simulink model "Dianlan_short"  (R2021a)
settings: Solver=VariableStepAuto  StartTime=0.0  StopTime=20e-6  RelTol=1e-3
libraries: spsGroundLib x4, spsVoltageMeasurementLib x3, spsDistributedParametersLineLib x2, spsSeriesRLCBranchLib x2, spsControlledVoltageSourceLib x1, spspowerguiLib x1
settings Model: Creator=张瑞  LastModifiedBy=张瑞

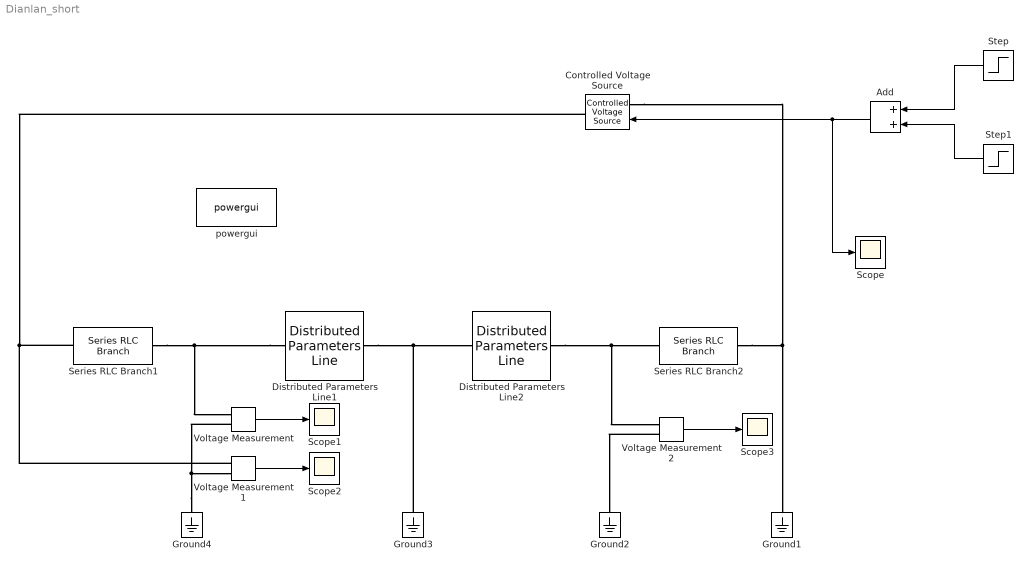
== system Dianlan_short ==
  Add : Sum
  Controlled Voltage Source : spsControlledVoltageSourceLib/Controlled Voltage Source  Initialize=off  Source_Type=AC  Amplitude=0  Phase=0  Frequency=0  Measurements=Voltage
  Distributed Parameters Line1 : spsDistributedParametersLineLib/Distributed Parameters Line  Phases=1  Length=1  Frequency=1000  Resistance=1.8E-1  Inductance=2.75E-4  Capacitance=5.57E-7  x1=[-1.238e-05 0;-1.237e-05 0;-1.236e-05 0;-1.235e-05 0;-1.234e-05 0;-1.233e-05 0;-1.232e-05 0;-1.231e-05 0;-1.23e-05 0;-1.229e-05 0;-1.228e-05 0;-1.227e-05 0;-1.226e-05 0;-1.225e-05 0;-1.224e-05 0;-1.223e-05 0;-1.222e-05 0;-1.221e-05 0;-1.22e-05 0;-1.219e-05 0;-1.218e-05 0;-1.217e-05 0;-1.216e-05 0;-1.215e-05 0;-1.214e-05 0;-1.213e-05 0;-1.212e-05 0;-1.211e-05 0;-1.21e-05 0;-1.209e-05 0;-1.208e-05 0;-1.207e-05 0;-1.206e-05 0;-1.205e-05 0;-1.204e-05 0;-1.203e-05 0;-1.202e-05 0;-1.201e-05 0;-1.2e-05 0;-1.199e-05 0;-1.198e-05 0;-1.197e-05 0;-1.196e-05 0;-1.195e-05 0;-1.194e-05 0;-1.193e-05 0;-1.192e-05 0;-1.191e-05 0;-1.19e-05 0;-1.189e-05 0;-1.188e-05 0;-1.187e-05 0;-1.186e-05 0;-1.185e-05 0;-1.184e-05 0;-1.183e-05 0;-1.182e-05 0;-1.181e-05 0;-1.18e-05 0;-1.179e-05 0;-1.178e-05 0;-1.177e-05 0;-1.176e-05 0;-1.175e-05 0;-1.174e-05 0;-1.173e-05 0;-1.172e-05 0;-1.171e-05 0;-1.17e-05 0;-1.169e-05 0;-1.168e-05 0;-1.167e-05 0;-1.166e-05 0;-1.165e-05 0;-1.164e-05 0;-1.163e-05 0;-1.162e-05 0;-1.161e-05 0;-1.16e-05 0;-1.159e-05 0;-1.158e-05 0;-1.157e-05 0;-1.156e-05 0;-1.155e-05 0;-1.154e-05 0;-1.153e-05 0;-1.152e-05 0;-1.151e-05 0;-1.15e-05 0;-1.149e-05 0;-1.148e-05 0;-1.147e-05 0;-1.146e-05 0;-1.145e-05 0;-1.144e-05 0;-1.143e-05 0;-1.142e-05 0;-1.141e-05 0;-1.14e-05 0;-1.139e-05 0;-1.138e-05 0;-1.137e-05 0;-1.136e-05 0;-1.135e-05 0;-1.134e-05 0;-1.133e-05 0;-1.132e-05 0;-1.131e-05 0;-1.13e-05 0;-1.129e-05 0;-1.128e-05 0;-1.127e-05 0;-1.126e-05 0;-1.125e-05 0;-1.124e-05 0;-1.123e-05 0;-1.122e-05 0;-1.121e-05 0;-1.12e-05 0;-1.119e-05 0;-1.118e-05 0;-1.117e-05 0;-1.116e-05 0;-1.115e-05 0;-1.114e-05 0;-1.113e-05 0;-1.112e-05 0;-1.111e-05 0;-1.11e-05 0;-1.109e-05 0;-1.108e-05 0;-1.107e-05 0;-1.106e-05 0;-1.105e-05 0;-1.104e-05 0;-1.103e-05 0;-1.102e-05 0;-1.101e-05 0;-1.1e-05 0;-1.099e-05 0;-1.098e-05 0;-1.097e-05 0;-1.096e-05 0;-1.095e-05 0;-1.094e-05 0;-1.093e-05 0;-1.092e-05 0;-1.091e-05 0;-1.09e-05 0;-1.089e-05 0;-1.088e-05 0;-1.087e-05 0;-1.086e-05 0;-1.085e-05 0;-1.084e-05 0;-1.083e-05 0;-1.082e-05 0;-1.081e-05 0;-1.08e-05 0;-1.079e-05 0;-1.078e-05 0;-1.077e-05 0;-1.076e-05 0;-1.075e-05 0;-1.074e-05 0;-1.073e-05 0;-1.072e-05 0;-1.071e-05 0;-1.07e-05 0;-1.069e-05 0;-1.068e-05 0;-1.067e-05 0;-1.066e-05 0;-1.065e-05 0;-1.064e-05 0;-1.063e-05 0;-1.062e-05 0;-1.061e-05 0;-1.06e-05 0;-1.059e-05 0;-1.058e-05 0;-1.057e-05 0;-1.056e-05 0;-1.055e-05 0;-1.054e-05 0;-1.053e-05 0;-1.052e-05 0;-1.051e-05 0;-1.05e-05 0;-1.049e-05 0;-1.048e-05 0;-1.047e-05 0;-1.046e-05 0;-1.045e-05 0;-1.044e-05 0;-1.043e-05 0;-1.042e-05 0;-1.041e-05 0;-1.04e-05 0;-1.039e-05 0;-1.038e-05 0;-1.037e-05 0;-1.036e-05 0;-1.035e-05 0;-1.034e-05 0;-1.033e-05 0;-1.032e-05 0;-1.031e-05 0;-1.03e-05 0;-1.029e-05 0;-1.028e-05 0;-1.027e-05 0;-1.026e-05 0;-1.025e-05 0;-1.024e-05 0;-1.023e-05 0;-1.022e-05 0;-1.021e-05 0;-1.02e-05 0;-1.019e-05 0;-1.018e-05 0;-1.017e-05 0;-1.016e-05 0;-1.015e-05 0;-1.014e-05 0;-1.013e-05 0;-1.012e-05 0;-1.011e-05 0;-1.01e-05 0;-1.009e-05 0;-1.008e-05 0;-1.007e-05 0;-1.006e-05 0;-1.005e-05 0;-1.004e-05 0;-1.003e-05 0;-1.002e-05 0;-1.001e-05 0;-1e-05 0;-9.99e-06 0;-9.98e-06 0;-9.97e-06 0;-9.96e-06 0;-9.95e-06 0;-9.94e-06 0;-9.93e-06 0;-9.92e-06 0;-9.91e-06 0;-9.9e-06 0;-9.89e-06 0;-9.88e-06 0;-9.87e-06 0;-9.86e-06 0;-9.85e-06 0;-9.84e-06 0;-9.83e-06 0;-9.82e-06 0;-9.81e-06 0;-9.8e-06 0;-9.79e-06 0;-9.78e-06 0;-9.77e-06 0;-9.76e-06 0;-9.75e-06 0;-9.74e-06 0;-9.73e-06 0;-9.72e-06 0;-9.71e-06 0;-9.7e-06 0;-9.69e-06 0;-9.68e-06 0;-9.67e-06 0;-9.66e-06 0;-9.65e-06 0;-9.64e-06 0;-9.63e-06 0;-9.62e-06 0;-9.61e-06 0;-9.6e-06 0;-9.59e-06 0;-9.58e-06 0;-9.57e-06 0;-9.56e-06 0;-9.55e-06 0;-9.54e-06 0;-9.53e-06 0;-9.52e-06 0;-9.51e-06 0;-9.5e-06 0;-9.49e-06 0;-9.48e-06 0;-9.47e-06 0;-9.46e-06 0;-9.45e-06 0;-9.44e-06 0;-9.43e-06 0;-9.42e-06 0;-9.41e-06 0;-9.4e-06 0;-9.39e-06 0;-9.38e-06 0;-9.37e-06 0;-9.36e-06 0;-9.35e-06 0;-9.34e-06 0;-9.33e-06 0;-9.32e-06 0;-9.31e-06 0;-9.3e-06 0;-9.29e-06 0;-9.28e-06 0;-9.27e-06 0;-9.26e-06 0;-9.25e-06 0;-9.24e-06 0;-9.23e-06 0 ...(+10828 chars)]  x2=[-1.238e-05 0;-1.237e-05 0;-1.236e-05 0;-1.235e-05 0;-1.234e-05 0;-1.233e-05 0;-1.232e-05 0;-1.231e-05 0;-1.23e-05 0;-1.229e-05 0;-1.228e-05 0;-1.227e-05 0;-1.226e-05 0;-1.225e-05 0;-1.224e-05 0;-1.223e-05 0;-1.222e-05 0;-1.221e-05 0;-1.22e-05 0;-1.219e-05 0;-1.218e-05 0;-1.217e-05 0;-1.216e-05 0;-1.215e-05 0;-1.214e-05 0;-1.213e-05 0;-1.212e-05 0;-1.211e-05 0;-1.21e-05 0;-1.209e-05 0;-1.208e-05 0;-1.207e-05 0;-1.206e-05 0;-1.205e-05 0;-1.204e-05 0;-1.203e-05 0;-1.202e-05 0;-1.201e-05 0;-1.2e-05 0;-1.199e-05 0;-1.198e-05 0;-1.197e-05 0;-1.196e-05 0;-1.195e-05 0;-1.194e-05 0;-1.193e-05 0;-1.192e-05 0;-1.191e-05 0;-1.19e-05 0;-1.189e-05 0;-1.188e-05 0;-1.187e-05 0;-1.186e-05 0;-1.185e-05 0;-1.184e-05 0;-1.183e-05 0;-1.182e-05 0;-1.181e-05 0;-1.18e-05 0;-1.179e-05 0;-1.178e-05 0;-1.177e-05 0;-1.176e-05 0;-1.175e-05 0;-1.174e-05 0;-1.173e-05 0;-1.172e-05 0;-1.171e-05 0;-1.17e-05 0;-1.169e-05 0;-1.168e-05 0;-1.167e-05 0;-1.166e-05 0;-1.165e-05 0;-1.164e-05 0;-1.163e-05 0;-1.162e-05 0;-1.161e-05 0;-1.16e-05 0;-1.159e-05 0;-1.158e-05 0;-1.157e-05 0;-1.156e-05 0;-1.155e-05 0;-1.154e-05 0;-1.153e-05 0;-1.152e-05 0;-1.151e-05 0;-1.15e-05 0;-1.149e-05 0;-1.148e-05 0;-1.147e-05 0;-1.146e-05 0;-1.145e-05 0;-1.144e-05 0;-1.143e-05 0;-1.142e-05 0;-1.141e-05 0;-1.14e-05 0;-1.139e-05 0;-1.138e-05 0;-1.137e-05 0;-1.136e-05 0;-1.135e-05 0;-1.134e-05 0;-1.133e-05 0;-1.132e-05 0;-1.131e-05 0;-1.13e-05 0;-1.129e-05 0;-1.128e-05 0;-1.127e-05 0;-1.126e-05 0;-1.125e-05 0;-1.124e-05 0;-1.123e-05 0;-1.122e-05 0;-1.121e-05 0;-1.12e-05 0;-1.119e-05 0;-1.118e-05 0;-1.117e-05 0;-1.116e-05 0;-1.115e-05 0;-1.114e-05 0;-1.113e-05 0;-1.112e-05 0;-1.111e-05 0;-1.11e-05 0;-1.109e-05 0;-1.108e-05 0;-1.107e-05 0;-1.106e-05 0;-1.105e-05 0;-1.104e-05 0;-1.103e-05 0;-1.102e-05 0;-1.101e-05 0;-1.1e-05 0;-1.099e-05 0;-1.098e-05 0;-1.097e-05 0;-1.096e-05 0;-1.095e-05 0;-1.094e-05 0;-1.093e-05 0;-1.092e-05 0;-1.091e-05 0;-1.09e-05 0;-1.089e-05 0;-1.088e-05 0;-1.087e-05 0;-1.086e-05 0;-1.085e-05 0;-1.084e-05 0;-1.083e-05 0;-1.082e-05 0;-1.081e-05 0;-1.08e-05 0;-1.079e-05 0;-1.078e-05 0;-1.077e-05 0;-1.076e-05 0;-1.075e-05 0;-1.074e-05 0;-1.073e-05 0;-1.072e-05 0;-1.071e-05 0;-1.07e-05 0;-1.069e-05 0;-1.068e-05 0;-1.067e-05 0;-1.066e-05 0;-1.065e-05 0;-1.064e-05 0;-1.063e-05 0;-1.062e-05 0;-1.061e-05 0;-1.06e-05 0;-1.059e-05 0;-1.058e-05 0;-1.057e-05 0;-1.056e-05 0;-1.055e-05 0;-1.054e-05 0;-1.053e-05 0;-1.052e-05 0;-1.051e-05 0;-1.05e-05 0;-1.049e-05 0;-1.048e-05 0;-1.047e-05 0;-1.046e-05 0;-1.045e-05 0;-1.044e-05 0;-1.043e-05 0;-1.042e-05 0;-1.041e-05 0;-1.04e-05 0;-1.039e-05 0;-1.038e-05 0;-1.037e-05 0;-1.036e-05 0;-1.035e-05 0;-1.034e-05 0;-1.033e-05 0;-1.032e-05 0;-1.031e-05 0;-1.03e-05 0;-1.029e-05 0;-1.028e-05 0;-1.027e-05 0;-1.026e-05 0;-1.025e-05 0;-1.024e-05 0;-1.023e-05 0;-1.022e-05 0;-1.021e-05 0;-1.02e-05 0;-1.019e-05 0;-1.018e-05 0;-1.017e-05 0;-1.016e-05 0;-1.015e-05 0;-1.014e-05 0;-1.013e-05 0;-1.012e-05 0;-1.011e-05 0;-1.01e-05 0;-1.009e-05 0;-1.008e-05 0;-1.007e-05 0;-1.006e-05 0;-1.005e-05 0;-1.004e-05 0;-1.003e-05 0;-1.002e-05 0;-1.001e-05 0;-1e-05 0;-9.99e-06 0;-9.98e-06 0;-9.97e-06 0;-9.96e-06 0;-9.95e-06 0;-9.94e-06 0;-9.93e-06 0;-9.92e-06 0;-9.91e-06 0;-9.9e-06 0;-9.89e-06 0;-9.88e-06 0;-9.87e-06 0;-9.86e-06 0;-9.85e-06 0;-9.84e-06 0;-9.83e-06 0;-9.82e-06 0;-9.81e-06 0;-9.8e-06 0;-9.79e-06 0;-9.78e-06 0;-9.77e-06 0;-9.76e-06 0;-9.75e-06 0;-9.74e-06 0;-9.73e-06 0;-9.72e-06 0;-9.71e-06 0;-9.7e-06 0;-9.69e-06 0;-9.68e-06 0;-9.67e-06 0;-9.66e-06 0;-9.65e-06 0;-9.64e-06 0;-9.63e-06 0;-9.62e-06 0;-9.61e-06 0;-9.6e-06 0;-9.59e-06 0;-9.58e-06 0;-9.57e-06 0;-9.56e-06 0;-9.55e-06 0;-9.54e-06 0;-9.53e-06 0;-9.52e-06 0;-9.51e-06 0;-9.5e-06 0;-9.49e-06 0;-9.48e-06 0;-9.47e-06 0;-9.46e-06 0;-9.45e-06 0;-9.44e-06 0;-9.43e-06 0;-9.42e-06 0;-9.41e-06 0;-9.4e-06 0;-9.39e-06 0;-9.38e-06 0;-9.37e-06 0;-9.36e-06 0;-9.35e-06 0;-9.34e-06 0;-9.33e-06 0;-9.32e-06 0;-9.31e-06 0;-9.3e-06 0;-9.29e-06 0;-9.28e-06 0;-9.27e-06 0;-9.26e-06 0;-9.25e-06 0;-9.24e-06 0;-9.23e-06 0 ...(+10828 chars)]  x3=[-1.238e-05 0;-1.237e-05 0;-1.236e-05 0;-1.235e-05 0;-1.234e-05 0;-1.233e-05 0;-1.232e-05 0;-1.231e-05 0;-1.23e-05 0;-1.229e-05 0;-1.228e-05 0;-1.227e-05 0;-1.226e-05 0;-1.225e-05 0;-1.224e-05 0;-1.223e-05 0;-1.222e-05 0;-1.221e-05 0;-1.22e-05 0;-1.219e-05 0;-1.218e-05 0;-1.217e-05 0;-1.216e-05 0;-1.215e-05 0;-1.214e-05 0;-1.213e-05 0;-1.212e-05 0;-1.211e-05 0;-1.21e-05 0;-1.209e-05 0;-1.208e-05 0;-1.207e-05 0;-1.206e-05 0;-1.205e-05 0;-1.204e-05 0;-1.203e-05 0;-1.202e-05 0;-1.201e-05 0;-1.2e-05 0;-1.199e-05 0;-1.198e-05 0;-1.197e-05 0;-1.196e-05 0;-1.195e-05 0;-1.194e-05 0;-1.193e-05 0;-1.192e-05 0;-1.191e-05 0;-1.19e-05 0;-1.189e-05 0;-1.188e-05 0;-1.187e-05 0;-1.186e-05 0;-1.185e-05 0;-1.184e-05 0;-1.183e-05 0;-1.182e-05 0;-1.181e-05 0;-1.18e-05 0;-1.179e-05 0;-1.178e-05 0;-1.177e-05 0;-1.176e-05 0;-1.175e-05 0;-1.174e-05 0;-1.173e-05 0;-1.172e-05 0;-1.171e-05 0;-1.17e-05 0;-1.169e-05 0;-1.168e-05 0;-1.167e-05 0;-1.166e-05 0;-1.165e-05 0;-1.164e-05 0;-1.163e-05 0;-1.162e-05 0;-1.161e-05 0;-1.16e-05 0;-1.159e-05 0;-1.158e-05 0;-1.157e-05 0;-1.156e-05 0;-1.155e-05 0;-1.154e-05 0;-1.153e-05 0;-1.152e-05 0;-1.151e-05 0;-1.15e-05 0;-1.149e-05 0;-1.148e-05 0;-1.147e-05 0;-1.146e-05 0;-1.145e-05 0;-1.144e-05 0;-1.143e-05 0;-1.142e-05 0;-1.141e-05 0;-1.14e-05 0;-1.139e-05 0;-1.138e-05 0;-1.137e-05 0;-1.136e-05 0;-1.135e-05 0;-1.134e-05 0;-1.133e-05 0;-1.132e-05 0;-1.131e-05 0;-1.13e-05 0;-1.129e-05 0;-1.128e-05 0;-1.127e-05 0;-1.126e-05 0;-1.125e-05 0;-1.124e-05 0;-1.123e-05 0;-1.122e-05 0;-1.121e-05 0;-1.12e-05 0;-1.119e-05 0;-1.118e-05 0;-1.117e-05 0;-1.116e-05 0;-1.115e-05 0;-1.114e-05 0;-1.113e-05 0;-1.112e-05 0;-1.111e-05 0;-1.11e-05 0;-1.109e-05 0;-1.108e-05 0;-1.107e-05 0;-1.106e-05 0;-1.105e-05 0;-1.104e-05 0;-1.103e-05 0;-1.102e-05 0;-1.101e-05 0;-1.1e-05 0;-1.099e-05 0;-1.098e-05 0;-1.097e-05 0;-1.096e-05 0;-1.095e-05 0;-1.094e-05 0;-1.093e-05 0;-1.092e-05 0;-1.091e-05 0;-1.09e-05 0;-1.089e-05 0;-1.088e-05 0;-1.087e-05 0;-1.086e-05 0;-1.085e-05 0;-1.084e-05 0;-1.083e-05 0;-1.082e-05 0;-1.081e-05 0;-1.08e-05 0;-1.079e-05 0;-1.078e-05 0;-1.077e-05 0;-1.076e-05 0;-1.075e-05 0;-1.074e-05 0;-1.073e-05 0;-1.072e-05 0;-1.071e-05 0;-1.07e-05 0;-1.069e-05 0;-1.068e-05 0;-1.067e-05 0;-1.066e-05 0;-1.065e-05 0;-1.064e-05 0;-1.063e-05 0;-1.062e-05 0;-1.061e-05 0;-1.06e-05 0;-1.059e-05 0;-1.058e-05 0;-1.057e-05 0;-1.056e-05 0;-1.055e-05 0;-1.054e-05 0;-1.053e-05 0;-1.052e-05 0;-1.051e-05 0;-1.05e-05 0;-1.049e-05 0;-1.048e-05 0;-1.047e-05 0;-1.046e-05 0;-1.045e-05 0;-1.044e-05 0;-1.043e-05 0;-1.042e-05 0;-1.041e-05 0;-1.04e-05 0;-1.039e-05 0;-1.038e-05 0;-1.037e-05 0;-1.036e-05 0;-1.035e-05 0;-1.034e-05 0;-1.033e-05 0;-1.032e-05 0;-1.031e-05 0;-1.03e-05 0;-1.029e-05 0;-1.028e-05 0;-1.027e-05 0;-1.026e-05 0;-1.025e-05 0;-1.024e-05 0;-1.023e-05 0;-1.022e-05 0;-1.021e-05 0;-1.02e-05 0;-1.019e-05 0;-1.018e-05 0;-1.017e-05 0;-1.016e-05 0;-1.015e-05 0;-1.014e-05 0;-1.013e-05 0;-1.012e-05 0;-1.011e-05 0;-1.01e-05 0;-1.009e-05 0;-1.008e-05 0;-1.007e-05 0;-1.006e-05 0;-1.005e-05 0;-1.004e-05 0;-1.003e-05 0;-1.002e-05 0;-1.001e-05 0;-1e-05 0;-9.99e-06 0;-9.98e-06 0;-9.97e-06 0;-9.96e-06 0;-9.95e-06 0;-9.94e-06 0;-9.93e-06 0;-9.92e-06 0;-9.91e-06 0;-9.9e-06 0;-9.89e-06 0;-9.88e-06 0;-9.87e-06 0;-9.86e-06 0;-9.85e-06 0;-9.84e-06 0;-9.83e-06 0;-9.82e-06 0;-9.81e-06 0;-9.8e-06 0;-9.79e-06 0;-9.78e-06 0;-9.77e-06 0;-9.76e-06 0;-9.75e-06 0;-9.74e-06 0;-9.73e-06 0;-9.72e-06 0;-9.71e-06 0;-9.7e-06 0;-9.69e-06 0;-9.68e-06 0;-9.67e-06 0;-9.66e-06 0;-9.65e-06 0;-9.64e-06 0;-9.63e-06 0;-9.62e-06 0;-9.61e-06 0;-9.6e-06 0;-9.59e-06 0;-9.58e-06 0;-9.57e-06 0;-9.56e-06 0;-9.55e-06 0;-9.54e-06 0;-9.53e-06 0;-9.52e-06 0;-9.51e-06 0;-9.5e-06 0;-9.49e-06 0;-9.48e-06 0;-9.47e-06 0;-9.46e-06 0;-9.45e-06 0;-9.44e-06 0;-9.43e-06 0;-9.42e-06 0;-9.41e-06 0;-9.4e-06 0;-9.39e-06 0;-9.38e-06 0;-9.37e-06 0;-9.36e-06 0;-9.35e-06 0;-9.34e-06 0;-9.33e-06 0;-9.32e-06 0;-9.31e-06 0;-9.3e-06 0;-9.29e-06 0;-9.28e-06 0;-9.27e-06 0;-9.26e-06 0;-9.25e-06 0;-9.24e-06 0;-9.23e-06 0 ...(+10828 chars)]  x4=[-1.238e-05 0;-1.237e-05 0;-1.236e-05 0;-1.235e-05 0;-1.234e-05 0;-1.233e-05 0;-1.232e-05 0;-1.231e-05 0;-1.23e-05 0;-1.229e-05 0;-1.228e-05 0;-1.227e-05 0;-1.226e-05 0;-1.225e-05 0;-1.224e-05 0;-1.223e-05 0;-1.222e-05 0;-1.221e-05 0;-1.22e-05 0;-1.219e-05 0;-1.218e-05 0;-1.217e-05 0;-1.216e-05 0;-1.215e-05 0;-1.214e-05 0;-1.213e-05 0;-1.212e-05 0;-1.211e-05 0;-1.21e-05 0;-1.209e-05 0;-1.208e-05 0;-1.207e-05 0;-1.206e-05 0;-1.205e-05 0;-1.204e-05 0;-1.203e-05 0;-1.202e-05 0;-1.201e-05 0;-1.2e-05 0;-1.199e-05 0;-1.198e-05 0;-1.197e-05 0;-1.196e-05 0;-1.195e-05 0;-1.194e-05 0;-1.193e-05 0;-1.192e-05 0;-1.191e-05 0;-1.19e-05 0;-1.189e-05 0;-1.188e-05 0;-1.187e-05 0;-1.186e-05 0;-1.185e-05 0;-1.184e-05 0;-1.183e-05 0;-1.182e-05 0;-1.181e-05 0;-1.18e-05 0;-1.179e-05 0;-1.178e-05 0;-1.177e-05 0;-1.176e-05 0;-1.175e-05 0;-1.174e-05 0;-1.173e-05 0;-1.172e-05 0;-1.171e-05 0;-1.17e-05 0;-1.169e-05 0;-1.168e-05 0;-1.167e-05 0;-1.166e-05 0;-1.165e-05 0;-1.164e-05 0;-1.163e-05 0;-1.162e-05 0;-1.161e-05 0;-1.16e-05 0;-1.159e-05 0;-1.158e-05 0;-1.157e-05 0;-1.156e-05 0;-1.155e-05 0;-1.154e-05 0;-1.153e-05 0;-1.152e-05 0;-1.151e-05 0;-1.15e-05 0;-1.149e-05 0;-1.148e-05 0;-1.147e-05 0;-1.146e-05 0;-1.145e-05 0;-1.144e-05 0;-1.143e-05 0;-1.142e-05 0;-1.141e-05 0;-1.14e-05 0;-1.139e-05 0;-1.138e-05 0;-1.137e-05 0;-1.136e-05 0;-1.135e-05 0;-1.134e-05 0;-1.133e-05 0;-1.132e-05 0;-1.131e-05 0;-1.13e-05 0;-1.129e-05 0;-1.128e-05 0;-1.127e-05 0;-1.126e-05 0;-1.125e-05 0;-1.124e-05 0;-1.123e-05 0;-1.122e-05 0;-1.121e-05 0;-1.12e-05 0;-1.119e-05 0;-1.118e-05 0;-1.117e-05 0;-1.116e-05 0;-1.115e-05 0;-1.114e-05 0;-1.113e-05 0;-1.112e-05 0;-1.111e-05 0;-1.11e-05 0;-1.109e-05 0;-1.108e-05 0;-1.107e-05 0;-1.106e-05 0;-1.105e-05 0;-1.104e-05 0;-1.103e-05 0;-1.102e-05 0;-1.101e-05 0;-1.1e-05 0;-1.099e-05 0;-1.098e-05 0;-1.097e-05 0;-1.096e-05 0;-1.095e-05 0;-1.094e-05 0;-1.093e-05 0;-1.092e-05 0;-1.091e-05 0;-1.09e-05 0;-1.089e-05 0;-1.088e-05 0;-1.087e-05 0;-1.086e-05 0;-1.085e-05 0;-1.084e-05 0;-1.083e-05 0;-1.082e-05 0;-1.081e-05 0;-1.08e-05 0;-1.079e-05 0;-1.078e-05 0;-1.077e-05 0;-1.076e-05 0;-1.075e-05 0;-1.074e-05 0;-1.073e-05 0;-1.072e-05 0;-1.071e-05 0;-1.07e-05 0;-1.069e-05 0;-1.068e-05 0;-1.067e-05 0;-1.066e-05 0;-1.065e-05 0;-1.064e-05 0;-1.063e-05 0;-1.062e-05 0;-1.061e-05 0;-1.06e-05 0;-1.059e-05 0;-1.058e-05 0;-1.057e-05 0;-1.056e-05 0;-1.055e-05 0;-1.054e-05 0;-1.053e-05 0;-1.052e-05 0;-1.051e-05 0;-1.05e-05 0;-1.049e-05 0;-1.048e-05 0;-1.047e-05 0;-1.046e-05 0;-1.045e-05 0;-1.044e-05 0;-1.043e-05 0;-1.042e-05 0;-1.041e-05 0;-1.04e-05 0;-1.039e-05 0;-1.038e-05 0;-1.037e-05 0;-1.036e-05 0;-1.035e-05 0;-1.034e-05 0;-1.033e-05 0;-1.032e-05 0;-1.031e-05 0;-1.03e-05 0;-1.029e-05 0;-1.028e-05 0;-1.027e-05 0;-1.026e-05 0;-1.025e-05 0;-1.024e-05 0;-1.023e-05 0;-1.022e-05 0;-1.021e-05 0;-1.02e-05 0;-1.019e-05 0;-1.018e-05 0;-1.017e-05 0;-1.016e-05 0;-1.015e-05 0;-1.014e-05 0;-1.013e-05 0;-1.012e-05 0;-1.011e-05 0;-1.01e-05 0;-1.009e-05 0;-1.008e-05 0;-1.007e-05 0;-1.006e-05 0;-1.005e-05 0;-1.004e-05 0;-1.003e-05 0;-1.002e-05 0;-1.001e-05 0;-1e-05 0;-9.99e-06 0;-9.98e-06 0;-9.97e-06 0;-9.96e-06 0;-9.95e-06 0;-9.94e-06 0;-9.93e-06 0;-9.92e-06 0;-9.91e-06 0;-9.9e-06 0;-9.89e-06 0;-9.88e-06 0;-9.87e-06 0;-9.86e-06 0;-9.85e-06 0;-9.84e-06 0;-9.83e-06 0;-9.82e-06 0;-9.81e-06 0;-9.8e-06 0;-9.79e-06 0;-9.78e-06 0;-9.77e-06 0;-9.76e-06 0;-9.75e-06 0;-9.74e-06 0;-9.73e-06 0;-9.72e-06 0;-9.71e-06 0;-9.7e-06 0;-9.69e-06 0;-9.68e-06 0;-9.67e-06 0;-9.66e-06 0;-9.65e-06 0;-9.64e-06 0;-9.63e-06 0;-9.62e-06 0;-9.61e-06 0;-9.6e-06 0;-9.59e-06 0;-9.58e-06 0;-9.57e-06 0;-9.56e-06 0;-9.55e-06 0;-9.54e-06 0;-9.53e-06 0;-9.52e-06 0;-9.51e-06 0;-9.5e-06 0;-9.49e-06 0;-9.48e-06 0;-9.47e-06 0;-9.46e-06 0;-9.45e-06 0;-9.44e-06 0;-9.43e-06 0;-9.42e-06 0;-9.41e-06 0;-9.4e-06 0;-9.39e-06 0;-9.38e-06 0;-9.37e-06 0;-9.36e-06 0;-9.35e-06 0;-9.34e-06 0;-9.33e-06 0;-9.32e-06 0;-9.31e-06 0;-9.3e-06 0;-9.29e-06 0;-9.28e-06 0;-9.27e-06 0;-9.26e-06 0;-9.25e-06 0;-9.24e-06 0;-9.23e-06 0 ...(+10828 chars)]  x5=1.23763888109577e-05  V1=ones(3,3)  V2=ones(3,3)  I1=ones(3,3)  I2=ones(3,3)  nHarmo=1  Measurements=Phase-to-ground voltages  Decoupling=off  VsMag0=0  VrMag0=0  VsAngle0=0  VrAngle0=0  IsMag0=0  IrMag0=0  IsAngle0=0  IrAngle0=0
      settings: SourceProductBaseCode=PS
  Distributed Parameters Line2 : spsDistributedParametersLineLib/Distributed Parameters Line  Phases=1  Length=0.2  Frequency=1000  Resistance=1.8E-1  Inductance=2.75E-4  Capacitance=5.57E-7  x1=[-2.48e-06 0;-2.47e-06 0;-2.46e-06 0;-2.45e-06 0;-2.44e-06 0;-2.43e-06 0;-2.42e-06 0;-2.41e-06 0;-2.4e-06 0;-2.39e-06 0;-2.38e-06 0;-2.37e-06 0;-2.36e-06 0;-2.35e-06 0;-2.34e-06 0;-2.33e-06 0;-2.32e-06 0;-2.31e-06 0;-2.3e-06 0;-2.29e-06 0;-2.28e-06 0;-2.27e-06 0;-2.26e-06 0;-2.25e-06 0;-2.24e-06 0;-2.23e-06 0;-2.22e-06 0;-2.21e-06 0;-2.2e-06 0;-2.19e-06 0;-2.18e-06 0;-2.17e-06 0;-2.16e-06 0;-2.15e-06 0;-2.14e-06 0;-2.13e-06 0;-2.12e-06 0;-2.11e-06 0;-2.1e-06 0;-2.09e-06 0;-2.08e-06 0;-2.07e-06 0;-2.06e-06 0;-2.05e-06 0;-2.04e-06 0;-2.03e-06 0;-2.02e-06 0;-2.01e-06 0;-2e-06 0;-1.99e-06 0;-1.98e-06 0;-1.97e-06 0;-1.96e-06 0;-1.95e-06 0;-1.94e-06 0;-1.93e-06 0;-1.92e-06 0;-1.91e-06 0;-1.9e-06 0;-1.89e-06 0;-1.88e-06 0;-1.87e-06 0;-1.86e-06 0;-1.85e-06 0;-1.84e-06 0;-1.83e-06 0;-1.82e-06 0;-1.81e-06 0;-1.8e-06 0;-1.79e-06 0;-1.78e-06 0;-1.77e-06 0;-1.76e-06 0;-1.75e-06 0;-1.74e-06 0;-1.73e-06 0;-1.72e-06 0;-1.71e-06 0;-1.7e-06 0;-1.69e-06 0;-1.68e-06 0;-1.67e-06 0;-1.66e-06 0;-1.65e-06 0;-1.64e-06 0;-1.63e-06 0;-1.62e-06 0;-1.61e-06 0;-1.6e-06 0;-1.59e-06 0;-1.58e-06 0;-1.57e-06 0;-1.56e-06 0;-1.55e-06 0;-1.54e-06 0;-1.53e-06 0;-1.52e-06 0;-1.51e-06 0;-1.5e-06 0;-1.49e-06 0;-1.48e-06 0;-1.47e-06 0;-1.46e-06 0;-1.45e-06 0;-1.44e-06 0;-1.43e-06 0;-1.42e-06 0;-1.41e-06 0;-1.4e-06 0;-1.39e-06 0;-1.38e-06 0;-1.37e-06 0;-1.36e-06 0;-1.35e-06 0;-1.34e-06 0;-1.33e-06 0;-1.32e-06 0;-1.31e-06 0;-1.3e-06 0;-1.29e-06 0;-1.28e-06 0;-1.27e-06 0;-1.26e-06 0;-1.25e-06 0;-1.24e-06 0;-1.23e-06 0;-1.22e-06 0;-1.21e-06 0;-1.2e-06 0;-1.19e-06 0;-1.18e-06 0;-1.17e-06 0;-1.16e-06 0;-1.15e-06 0;-1.14e-06 0;-1.13e-06 0;-1.12e-06 0;-1.11e-06 0;-1.1e-06 0;-1.09e-06 0;-1.08e-06 0;-1.07e-06 0;-1.06e-06 0;-1.05e-06 0;-1.04e-06 0;-1.03e-06 0;-1.02e-06 0;-1.01e-06 0;-1e-06 0;-9.9e-07 0;-9.8e-07 0;-9.7e-07 0;-9.6e-07 0;-9.5e-07 0;-9.4e-07 0;-9.3e-07 0;-9.2e-07 0;-9.1e-07 0;-9e-07 0;-8.9e-07 0;-8.8e-07 0;-8.7e-07 0;-8.6e-07 0;-8.5e-07 0;-8.4e-07 0;-8.3e-07 0;-8.2e-07 0;-8.1e-07 0;-8e-07 0;-7.9e-07 0;-7.8e-07 0;-7.7e-07 0;-7.6e-07 0;-7.5e-07 0;-7.4e-07 0;-7.3e-07 0;-7.2e-07 0;-7.1e-07 0;-7e-07 0;-6.9e-07 0;-6.8e-07 0;-6.7e-07 0;-6.6e-07 0;-6.5e-07 0;-6.4e-07 0;-6.3e-07 0;-6.2e-07 0;-6.1e-07 0;-6e-07 0;-5.9e-07 0;-5.8e-07 0;-5.7e-07 0;-5.6e-07 0;-5.5e-07 0;-5.4e-07 0;-5.3e-07 0;-5.2e-07 0;-5.1e-07 0;-5e-07 0;-4.9e-07 0;-4.8e-07 0;-4.7e-07 0;-4.6e-07 0;-4.5e-07 0;-4.4e-07 0;-4.3e-07 0;-4.2e-07 0;-4.1e-07 0;-4e-07 0;-3.9e-07 0;-3.8e-07 0;-3.7e-07 0;-3.6e-07 0;-3.5e-07 0;-3.4e-07 0;-3.3e-07 0;-3.2e-07 0;-3.1e-07 0;-3e-07 0;-2.9e-07 0;-2.8e-07 0;-2.7e-07 0;-2.6e-07 0;-2.5e-07 0;-2.4e-07 0;-2.3e-07 0;-2.2e-07 0;-2.1e-07 0;-2e-07 0;-1.9e-07 0;-1.8e-07 0;-1.7e-07 0;-1.6e-07 0;-1.5e-07 0;-1.4e-07 0;-1.3e-07 0;-1.2e-07 0;-1.1e-07 0;-1e-07 0;-9e-08 0;-8e-08 0;-7e-08 0;-6e-08 0;-5e-08 0;-4e-08 0;-3e-08 0;-2e-08 0;-1e-08 0]  x2=[-2.48e-06 0;-2.47e-06 0;-2.46e-06 0;-2.45e-06 0;-2.44e-06 0;-2.43e-06 0;-2.42e-06 0;-2.41e-06 0;-2.4e-06 0;-2.39e-06 0;-2.38e-06 0;-2.37e-06 0;-2.36e-06 0;-2.35e-06 0;-2.34e-06 0;-2.33e-06 0;-2.32e-06 0;-2.31e-06 0;-2.3e-06 0;-2.29e-06 0;-2.28e-06 0;-2.27e-06 0;-2.26e-06 0;-2.25e-06 0;-2.24e-06 0;-2.23e-06 0;-2.22e-06 0;-2.21e-06 0;-2.2e-06 0;-2.19e-06 0;-2.18e-06 0;-2.17e-06 0;-2.16e-06 0;-2.15e-06 0;-2.14e-06 0;-2.13e-06 0;-2.12e-06 0;-2.11e-06 0;-2.1e-06 0;-2.09e-06 0;-2.08e-06 0;-2.07e-06 0;-2.06e-06 0;-2.05e-06 0;-2.04e-06 0;-2.03e-06 0;-2.02e-06 0;-2.01e-06 0;-2e-06 0;-1.99e-06 0;-1.98e-06 0;-1.97e-06 0;-1.96e-06 0;-1.95e-06 0;-1.94e-06 0;-1.93e-06 0;-1.92e-06 0;-1.91e-06 0;-1.9e-06 0;-1.89e-06 0;-1.88e-06 0;-1.87e-06 0;-1.86e-06 0;-1.85e-06 0;-1.84e-06 0;-1.83e-06 0;-1.82e-06 0;-1.81e-06 0;-1.8e-06 0;-1.79e-06 0;-1.78e-06 0;-1.77e-06 0;-1.76e-06 0;-1.75e-06 0;-1.74e-06 0;-1.73e-06 0;-1.72e-06 0;-1.71e-06 0;-1.7e-06 0;-1.69e-06 0;-1.68e-06 0;-1.67e-06 0;-1.66e-06 0;-1.65e-06 0;-1.64e-06 0;-1.63e-06 0;-1.62e-06 0;-1.61e-06 0;-1.6e-06 0;-1.59e-06 0;-1.58e-06 0;-1.57e-06 0;-1.56e-06 0;-1.55e-06 0;-1.54e-06 0;-1.53e-06 0;-1.52e-06 0;-1.51e-06 0;-1.5e-06 0;-1.49e-06 0;-1.48e-06 0;-1.47e-06 0;-1.46e-06 0;-1.45e-06 0;-1.44e-06 0;-1.43e-06 0;-1.42e-06 0;-1.41e-06 0;-1.4e-06 0;-1.39e-06 0;-1.38e-06 0;-1.37e-06 0;-1.36e-06 0;-1.35e-06 0;-1.34e-06 0;-1.33e-06 0;-1.32e-06 0;-1.31e-06 0;-1.3e-06 0;-1.29e-06 0;-1.28e-06 0;-1.27e-06 0;-1.26e-06 0;-1.25e-06 0;-1.24e-06 0;-1.23e-06 0;-1.22e-06 0;-1.21e-06 0;-1.2e-06 0;-1.19e-06 0;-1.18e-06 0;-1.17e-06 0;-1.16e-06 0;-1.15e-06 0;-1.14e-06 0;-1.13e-06 0;-1.12e-06 0;-1.11e-06 0;-1.1e-06 0;-1.09e-06 0;-1.08e-06 0;-1.07e-06 0;-1.06e-06 0;-1.05e-06 0;-1.04e-06 0;-1.03e-06 0;-1.02e-06 0;-1.01e-06 0;-1e-06 0;-9.9e-07 0;-9.8e-07 0;-9.7e-07 0;-9.6e-07 0;-9.5e-07 0;-9.4e-07 0;-9.3e-07 0;-9.2e-07 0;-9.1e-07 0;-9e-07 0;-8.9e-07 0;-8.8e-07 0;-8.7e-07 0;-8.6e-07 0;-8.5e-07 0;-8.4e-07 0;-8.3e-07 0;-8.2e-07 0;-8.1e-07 0;-8e-07 0;-7.9e-07 0;-7.8e-07 0;-7.7e-07 0;-7.6e-07 0;-7.5e-07 0;-7.4e-07 0;-7.3e-07 0;-7.2e-07 0;-7.1e-07 0;-7e-07 0;-6.9e-07 0;-6.8e-07 0;-6.7e-07 0;-6.6e-07 0;-6.5e-07 0;-6.4e-07 0;-6.3e-07 0;-6.2e-07 0;-6.1e-07 0;-6e-07 0;-5.9e-07 0;-5.8e-07 0;-5.7e-07 0;-5.6e-07 0;-5.5e-07 0;-5.4e-07 0;-5.3e-07 0;-5.2e-07 0;-5.1e-07 0;-5e-07 0;-4.9e-07 0;-4.8e-07 0;-4.7e-07 0;-4.6e-07 0;-4.5e-07 0;-4.4e-07 0;-4.3e-07 0;-4.2e-07 0;-4.1e-07 0;-4e-07 0;-3.9e-07 0;-3.8e-07 0;-3.7e-07 0;-3.6e-07 0;-3.5e-07 0;-3.4e-07 0;-3.3e-07 0;-3.2e-07 0;-3.1e-07 0;-3e-07 0;-2.9e-07 0;-2.8e-07 0;-2.7e-07 0;-2.6e-07 0;-2.5e-07 0;-2.4e-07 0;-2.3e-07 0;-2.2e-07 0;-2.1e-07 0;-2e-07 0;-1.9e-07 0;-1.8e-07 0;-1.7e-07 0;-1.6e-07 0;-1.5e-07 0;-1.4e-07 0;-1.3e-07 0;-1.2e-07 0;-1.1e-07 0;-1e-07 0;-9e-08 0;-8e-08 0;-7e-08 0;-6e-08 0;-5e-08 0;-4e-08 0;-3e-08 0;-2e-08 0;-1e-08 0]  x3=[-2.48e-06 0;-2.47e-06 0;-2.46e-06 0;-2.45e-06 0;-2.44e-06 0;-2.43e-06 0;-2.42e-06 0;-2.41e-06 0;-2.4e-06 0;-2.39e-06 0;-2.38e-06 0;-2.37e-06 0;-2.36e-06 0;-2.35e-06 0;-2.34e-06 0;-2.33e-06 0;-2.32e-06 0;-2.31e-06 0;-2.3e-06 0;-2.29e-06 0;-2.28e-06 0;-2.27e-06 0;-2.26e-06 0;-2.25e-06 0;-2.24e-06 0;-2.23e-06 0;-2.22e-06 0;-2.21e-06 0;-2.2e-06 0;-2.19e-06 0;-2.18e-06 0;-2.17e-06 0;-2.16e-06 0;-2.15e-06 0;-2.14e-06 0;-2.13e-06 0;-2.12e-06 0;-2.11e-06 0;-2.1e-06 0;-2.09e-06 0;-2.08e-06 0;-2.07e-06 0;-2.06e-06 0;-2.05e-06 0;-2.04e-06 0;-2.03e-06 0;-2.02e-06 0;-2.01e-06 0;-2e-06 0;-1.99e-06 0;-1.98e-06 0;-1.97e-06 0;-1.96e-06 0;-1.95e-06 0;-1.94e-06 0;-1.93e-06 0;-1.92e-06 0;-1.91e-06 0;-1.9e-06 0;-1.89e-06 0;-1.88e-06 0;-1.87e-06 0;-1.86e-06 0;-1.85e-06 0;-1.84e-06 0;-1.83e-06 0;-1.82e-06 0;-1.81e-06 0;-1.8e-06 0;-1.79e-06 0;-1.78e-06 0;-1.77e-06 0;-1.76e-06 0;-1.75e-06 0;-1.74e-06 0;-1.73e-06 0;-1.72e-06 0;-1.71e-06 0;-1.7e-06 0;-1.69e-06 0;-1.68e-06 0;-1.67e-06 0;-1.66e-06 0;-1.65e-06 0;-1.64e-06 0;-1.63e-06 0;-1.62e-06 0;-1.61e-06 0;-1.6e-06 0;-1.59e-06 0;-1.58e-06 0;-1.57e-06 0;-1.56e-06 0;-1.55e-06 0;-1.54e-06 0;-1.53e-06 0;-1.52e-06 0;-1.51e-06 0;-1.5e-06 0;-1.49e-06 0;-1.48e-06 0;-1.47e-06 0;-1.46e-06 0;-1.45e-06 0;-1.44e-06 0;-1.43e-06 0;-1.42e-06 0;-1.41e-06 0;-1.4e-06 0;-1.39e-06 0;-1.38e-06 0;-1.37e-06 0;-1.36e-06 0;-1.35e-06 0;-1.34e-06 0;-1.33e-06 0;-1.32e-06 0;-1.31e-06 0;-1.3e-06 0;-1.29e-06 0;-1.28e-06 0;-1.27e-06 0;-1.26e-06 0;-1.25e-06 0;-1.24e-06 0;-1.23e-06 0;-1.22e-06 0;-1.21e-06 0;-1.2e-06 0;-1.19e-06 0;-1.18e-06 0;-1.17e-06 0;-1.16e-06 0;-1.15e-06 0;-1.14e-06 0;-1.13e-06 0;-1.12e-06 0;-1.11e-06 0;-1.1e-06 0;-1.09e-06 0;-1.08e-06 0;-1.07e-06 0;-1.06e-06 0;-1.05e-06 0;-1.04e-06 0;-1.03e-06 0;-1.02e-06 0;-1.01e-06 0;-1e-06 0;-9.9e-07 0;-9.8e-07 0;-9.7e-07 0;-9.6e-07 0;-9.5e-07 0;-9.4e-07 0;-9.3e-07 0;-9.2e-07 0;-9.1e-07 0;-9e-07 0;-8.9e-07 0;-8.8e-07 0;-8.7e-07 0;-8.6e-07 0;-8.5e-07 0;-8.4e-07 0;-8.3e-07 0;-8.2e-07 0;-8.1e-07 0;-8e-07 0;-7.9e-07 0;-7.8e-07 0;-7.7e-07 0;-7.6e-07 0;-7.5e-07 0;-7.4e-07 0;-7.3e-07 0;-7.2e-07 0;-7.1e-07 0;-7e-07 0;-6.9e-07 0;-6.8e-07 0;-6.7e-07 0;-6.6e-07 0;-6.5e-07 0;-6.4e-07 0;-6.3e-07 0;-6.2e-07 0;-6.1e-07 0;-6e-07 0;-5.9e-07 0;-5.8e-07 0;-5.7e-07 0;-5.6e-07 0;-5.5e-07 0;-5.4e-07 0;-5.3e-07 0;-5.2e-07 0;-5.1e-07 0;-5e-07 0;-4.9e-07 0;-4.8e-07 0;-4.7e-07 0;-4.6e-07 0;-4.5e-07 0;-4.4e-07 0;-4.3e-07 0;-4.2e-07 0;-4.1e-07 0;-4e-07 0;-3.9e-07 0;-3.8e-07 0;-3.7e-07 0;-3.6e-07 0;-3.5e-07 0;-3.4e-07 0;-3.3e-07 0;-3.2e-07 0;-3.1e-07 0;-3e-07 0;-2.9e-07 0;-2.8e-07 0;-2.7e-07 0;-2.6e-07 0;-2.5e-07 0;-2.4e-07 0;-2.3e-07 0;-2.2e-07 0;-2.1e-07 0;-2e-07 0;-1.9e-07 0;-1.8e-07 0;-1.7e-07 0;-1.6e-07 0;-1.5e-07 0;-1.4e-07 0;-1.3e-07 0;-1.2e-07 0;-1.1e-07 0;-1e-07 0;-9e-08 0;-8e-08 0;-7e-08 0;-6e-08 0;-5e-08 0;-4e-08 0;-3e-08 0;-2e-08 0;-1e-08 0]  x4=[-2.48e-06 0;-2.47e-06 0;-2.46e-06 0;-2.45e-06 0;-2.44e-06 0;-2.43e-06 0;-2.42e-06 0;-2.41e-06 0;-2.4e-06 0;-2.39e-06 0;-2.38e-06 0;-2.37e-06 0;-2.36e-06 0;-2.35e-06 0;-2.34e-06 0;-2.33e-06 0;-2.32e-06 0;-2.31e-06 0;-2.3e-06 0;-2.29e-06 0;-2.28e-06 0;-2.27e-06 0;-2.26e-06 0;-2.25e-06 0;-2.24e-06 0;-2.23e-06 0;-2.22e-06 0;-2.21e-06 0;-2.2e-06 0;-2.19e-06 0;-2.18e-06 0;-2.17e-06 0;-2.16e-06 0;-2.15e-06 0;-2.14e-06 0;-2.13e-06 0;-2.12e-06 0;-2.11e-06 0;-2.1e-06 0;-2.09e-06 0;-2.08e-06 0;-2.07e-06 0;-2.06e-06 0;-2.05e-06 0;-2.04e-06 0;-2.03e-06 0;-2.02e-06 0;-2.01e-06 0;-2e-06 0;-1.99e-06 0;-1.98e-06 0;-1.97e-06 0;-1.96e-06 0;-1.95e-06 0;-1.94e-06 0;-1.93e-06 0;-1.92e-06 0;-1.91e-06 0;-1.9e-06 0;-1.89e-06 0;-1.88e-06 0;-1.87e-06 0;-1.86e-06 0;-1.85e-06 0;-1.84e-06 0;-1.83e-06 0;-1.82e-06 0;-1.81e-06 0;-1.8e-06 0;-1.79e-06 0;-1.78e-06 0;-1.77e-06 0;-1.76e-06 0;-1.75e-06 0;-1.74e-06 0;-1.73e-06 0;-1.72e-06 0;-1.71e-06 0;-1.7e-06 0;-1.69e-06 0;-1.68e-06 0;-1.67e-06 0;-1.66e-06 0;-1.65e-06 0;-1.64e-06 0;-1.63e-06 0;-1.62e-06 0;-1.61e-06 0;-1.6e-06 0;-1.59e-06 0;-1.58e-06 0;-1.57e-06 0;-1.56e-06 0;-1.55e-06 0;-1.54e-06 0;-1.53e-06 0;-1.52e-06 0;-1.51e-06 0;-1.5e-06 0;-1.49e-06 0;-1.48e-06 0;-1.47e-06 0;-1.46e-06 0;-1.45e-06 0;-1.44e-06 0;-1.43e-06 0;-1.42e-06 0;-1.41e-06 0;-1.4e-06 0;-1.39e-06 0;-1.38e-06 0;-1.37e-06 0;-1.36e-06 0;-1.35e-06 0;-1.34e-06 0;-1.33e-06 0;-1.32e-06 0;-1.31e-06 0;-1.3e-06 0;-1.29e-06 0;-1.28e-06 0;-1.27e-06 0;-1.26e-06 0;-1.25e-06 0;-1.24e-06 0;-1.23e-06 0;-1.22e-06 0;-1.21e-06 0;-1.2e-06 0;-1.19e-06 0;-1.18e-06 0;-1.17e-06 0;-1.16e-06 0;-1.15e-06 0;-1.14e-06 0;-1.13e-06 0;-1.12e-06 0;-1.11e-06 0;-1.1e-06 0;-1.09e-06 0;-1.08e-06 0;-1.07e-06 0;-1.06e-06 0;-1.05e-06 0;-1.04e-06 0;-1.03e-06 0;-1.02e-06 0;-1.01e-06 0;-1e-06 0;-9.9e-07 0;-9.8e-07 0;-9.7e-07 0;-9.6e-07 0;-9.5e-07 0;-9.4e-07 0;-9.3e-07 0;-9.2e-07 0;-9.1e-07 0;-9e-07 0;-8.9e-07 0;-8.8e-07 0;-8.7e-07 0;-8.6e-07 0;-8.5e-07 0;-8.4e-07 0;-8.3e-07 0;-8.2e-07 0;-8.1e-07 0;-8e-07 0;-7.9e-07 0;-7.8e-07 0;-7.7e-07 0;-7.6e-07 0;-7.5e-07 0;-7.4e-07 0;-7.3e-07 0;-7.2e-07 0;-7.1e-07 0;-7e-07 0;-6.9e-07 0;-6.8e-07 0;-6.7e-07 0;-6.6e-07 0;-6.5e-07 0;-6.4e-07 0;-6.3e-07 0;-6.2e-07 0;-6.1e-07 0;-6e-07 0;-5.9e-07 0;-5.8e-07 0;-5.7e-07 0;-5.6e-07 0;-5.5e-07 0;-5.4e-07 0;-5.3e-07 0;-5.2e-07 0;-5.1e-07 0;-5e-07 0;-4.9e-07 0;-4.8e-07 0;-4.7e-07 0;-4.6e-07 0;-4.5e-07 0;-4.4e-07 0;-4.3e-07 0;-4.2e-07 0;-4.1e-07 0;-4e-07 0;-3.9e-07 0;-3.8e-07 0;-3.7e-07 0;-3.6e-07 0;-3.5e-07 0;-3.4e-07 0;-3.3e-07 0;-3.2e-07 0;-3.1e-07 0;-3e-07 0;-2.9e-07 0;-2.8e-07 0;-2.7e-07 0;-2.6e-07 0;-2.5e-07 0;-2.4e-07 0;-2.3e-07 0;-2.2e-07 0;-2.1e-07 0;-2e-07 0;-1.9e-07 0;-1.8e-07 0;-1.7e-07 0;-1.6e-07 0;-1.5e-07 0;-1.4e-07 0;-1.3e-07 0;-1.2e-07 0;-1.1e-07 0;-1e-07 0;-9e-08 0;-8e-08 0;-7e-08 0;-6e-08 0;-5e-08 0;-4e-08 0;-3e-08 0;-2e-08 0;-1e-08 0]  x5=2.47527776219155e-06  V1=ones(3,3)  V2=ones(3,3)  I1=ones(3,3)  I2=ones(3,3)  nHarmo=1  Measurements=Phase-to-ground voltages  Decoupling=off  VsMag0=0  VrMag0=0  VsAngle0=0  VrAngle0=0  IsMag0=0  IrMag0=0  IsAngle0=0  IrAngle0=0
      settings: SourceProductBaseCode=PS
  Ground{1..4} (4 alike) : spsGroundLib/Ground  LConnTagsString=a
  Scope{,1..3} (4 alike) : Scope
  Series RLC Branch1 : spsSeriesRLCBranchLib/Series RLC Branch  LConnTagsString=__new0  RConnTagsString=__new0  BranchType=R  Resistance=1  Inductance=1e-3  SetiL0=off  InitialCurrent=0  Capacitance=1e-6  Setx0=off  InitialVoltage=0  Measurements=None
  Series RLC Branch2 : spsSeriesRLCBranchLib/Series RLC Branch  LConnTagsString=__new0  RConnTagsString=__new0  BranchType=R  Resistance=22.2  Inductance=1e-3  SetiL0=off  InitialCurrent=0  Capacitance=1e-6  Setx0=off  InitialVoltage=0  Measurements=None
  Step : Step  Time=0.3E-6  Before=28  After=0  SampleTime=1E-08
  Step1 : Step  Time=0.1E-6  Before=-28  After=0  SampleTime=1E-08
  Voltage Measurement : spsVoltageMeasurementLib/Voltage Measurement  PhasorSimulation=off  OutputType=Complex  PSBequivalent=0
  Voltage Measurement1 : spsVoltageMeasurementLib/Voltage Measurement  PhasorSimulation=off  OutputType=Complex  PSBequivalent=0
  Voltage Measurement2 : spsVoltageMeasurementLib/Voltage Measurement  PhasorSimulation=off  OutputType=Complex  PSBequivalent=0
  powergui : spspowerguiLib/powergui  Priority=1  SimulationMode=Discrete  SampleTime=0.01e-6  frequency=60  Iterations=50  frequencyindice=0  Pbase=100e6  ErrMax=1e-4  UnitsV=kV  UnitsW=MW  buscounter=0  FunctionMessages=off  echomessages=off  EnableUseOfTLC=off  CurrentSourceSwitches=off  DisableSnubberDevices=off  DisableRonSwitches=off  DisableVfSwitches=off  DisplayEquations=off  AutomaticDiscreteSolvers=off  SolverType=Tustin/Backward Euler (TBE)  Interpol=off  ExternalGateDelay=off  methode=off  Ts=100  x0status=blocks  SPID=on  SwTol=0  HookPort=off  NonlinearTolerance=1e-4  nMaxIteration=100  ContinueOnMaxIteration=off  RestoreLinks=warning  ResistiveCurrentMeasurement=off  Frange=[0:2:500]  Ylog=off  Xlog=on  ShowGrid=off  save=off  variable=ZData  structure=0  ZoomFFT=off  StartTime=0.0  cycles=1  DisplayStyle=1  fundamental=60  FreqAxis=off  MaxFrequency=1000  frequencyindicesteady=1  RmsSteady=1  display=off
  wires:
  Voltage Measurement/1 -> Scope1/1
  Voltage Measurement1/1 -> Scope2/1
  Voltage Measurement2/1 -> Scope3/1
  Add/1 -> Scope/1, Controlled Voltage Source/1
  Step/1 -> Add/1
  Step1/1 -> Add/2
  connections:
  Controlled Voltage Source/RConn1 -- Voltage Measurement1/LConn1 -- Series RLC Branch1/LConn1
  Distributed Parameters Line1/LConn1 -- Series RLC Branch1/RConn1 -- Voltage Measurement/LConn1
  Distributed Parameters Line2/RConn1 -- Voltage Measurement2/LConn1 -- Series RLC Branch2/LConn1
  Series RLC Branch2/RConn1 -- Ground1/LConn1 -- Controlled Voltage Source/LConn1
  Voltage Measurement2/LConn2 -- Ground2/LConn1
  Ground4/LConn1 -- Voltage Measurement/LConn2 -- Voltage Measurement1/LConn2
  Distributed Parameters Line1/RConn1 -- Distributed Parameters Line2/LConn1 -- Ground3/LConn1
